simulink model "pacemaker_Integrated_modes_updated_AAI_VVI"  (R2023b)
settings: Solver=FixedStepAuto  StartTime=0.0  StopTime=10  FixedStep=1e-3  RelTol=1e-3  EnableMultiTasking=on
undefined symbols (not defined in the file): D0, D1, D10, D11, D12, D13, D2, D3, D4, D5, D6, D7, D8, D9, PTA0, PTA1, PTA2, PTB23, PTB9, PTC16, PTC17, PTC2, PTC3, PTC4, PTD0, PTD1, PTD2, PTD3
libraries: frdmk64flib x16
settings Model: ExtModeTrigDuration=5  Creator=sadeg  LastModifiedBy=ayush
settings OptimizationCC: EnhancedBackFolding=on  PassReuseOutputArgsThreshold=0  MaxStackSize=64  OptimizeBlockOrder=speed  DifferentSizesBufferReuse=on  OptimizationCustomize=off
settings DebuggingCC: ParameterTunabilityLossMsg=error
settings HardwareCC: ProdBitPerPointer=32  ProdBitPerSizeT=32  ProdBitPerPtrDiffT=32  ProdLargestAtomicInteger=Long  ProdLargestAtomicFloat=Double  ProdWordSize=32  ProdHWDeviceType=ARM Compatible->ARM Cortex  UseEmbeddedCoderFeatures=off
settings SFSimCC: MATLABDynamicMemAlloc=off
settings RTWCC: Description=Embedded Coder  SystemTargetFile=ert.tlc  HardwareBoard=NXP FRDM-K64F  TLCOptions="-aInlineSetEventsForThisBaseRateFcn=TLC_FALSE -aSuppressMultiTaskScheduler=TLC_FALSE  -aRateBasedStepFcn=0"  TemplateMakefile=ert_default_tmf  Toolchain=GNU Tools for ARM Embedded Processors
settings CodeAppCC: ForceParamTrailComments=on  OperatorAnnotations=on
settings ERTTargetCC: ERTCustomFileBanners=off  SupportContinuousTime=on  SupportNonInlinedSFcns=on  RemoveResetFunc=off  ModelStepFunctionPrototypeControlCompliant=off  ExtModeTransport=4  ExtModeMexFile=sendToCommService

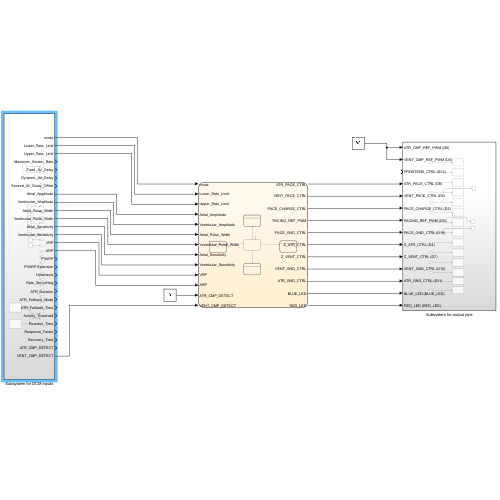
[thumbnail: Simulink's stored preview of the top-level diagram]
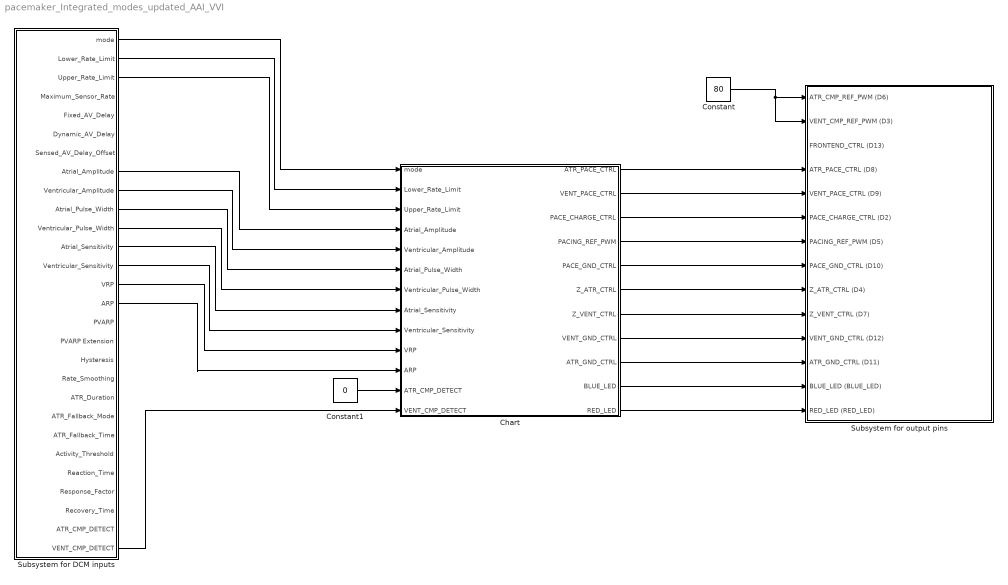
== system pacemaker_Integrated_modes_updated_AAI_VVI ==
  Chart : Stateflow chart  TreatAsAtomicUnit=on
      settings: PortSchema="{\"entries\":[{\"content\":{\"sides\":[{\"content\":{\"connectorIds\":[\"In13\",\"In1\",\"In2\",\"In3\",\"In5\",\"In4\",\"In6\",\"In7\",\"In8\",\"In10\",\"In9\",\"In12\",\"In11\"]},\"type\":\"ConnectorPlacement.EquallySpacedRectSide\",\"uuid\":\"4624e3e5-9266-4e51-8f1f-a7517f1382a8\"},{\"content\":{\"connectorIds\":[\"Out3\",\"Out4\",\"Out2\",\"Out5\",\"Out6\",\"Out7\",\"Out1\",\"Out8\",\"Out9\",\"Out10\",\"Out11\"],\"side\":\"RIGHT\"},\"type\":\"ConnectorPlacement.EquallySpacedRectSide\",\"uuid\":\"506810c9-9779-465d-935e-bf5d90de1bf6\"},{\"content\":{\"side\":\"TOP\"},\"type\":\"ConnectorPlacement.EquallySpacedRectSide\",\"uuid\":\"ef5dabc6-fa85-4901-94e2-5ef8203e9e04\"}]},\"type\":\"ConnectorPlacement.EquallySpacedConnector\",\"uuid\":\"5b51df89-7be9-413b-8f7d-b7db43a61802\"}],\"packageUris\":[\"http://schema.mathworks.com/mf0/Connector/R2020b\"],\"version\":\"1.0\"}"
  Constant : Constant  Value=80
  Constant1 : Constant  Value=0
  Subsystem for DCM inputs : Subsystem
  Subsystem for output pins : Subsystem
  wires:
  Constant/1 -> Subsystem for output pins/2(VENT_CMP_REF_PWM (D3)), Subsystem for output pins/1(ATR_CMP_REF_PWM (D6))
  Subsystem for DCM inputs/2(Lower_Rate_Limit) -> Chart/1(Lower_Rate_Limit)
  Subsystem for DCM inputs/3(Upper_Rate_Limit) -> Chart/2(Upper_Rate_Limit)
  Subsystem for DCM inputs/8(Atrial_Amplitude) -> Chart/3(Atrial_Amplitude)
  Subsystem for DCM inputs/10(Atrial_Pulse_Width) -> Chart/4(Atrial_Pulse_Width)
  Subsystem for DCM inputs/9(Ventricular_Amplitude) -> Chart/5(Ventricular_Amplitude)
  Subsystem for DCM inputs/11(Ventricular_Pulse_Width) -> Chart/6(Ventricular_Pulse_Width)
  Subsystem for DCM inputs/12(Atrial_Sensitivity) -> Chart/7(Atrial_Sensitivity)
  Subsystem for DCM inputs/13(Ventricular_Sensitivity) -> Chart/8(Ventricular_Sensitivity)
  Subsystem for DCM inputs/15(ARP) -> Chart/9(ARP)
  Subsystem for DCM inputs/14(VRP) -> Chart/10(VRP)
  Chart/1(Z_VENT_CTRL) -> Subsystem for output pins/10(Z_VENT_CTRL (D7))
  Chart/2(PACE_CHARGE_CTRL) -> Subsystem for output pins/6(PACE_CHARGE_CTRL (D2))
  Chart/3(ATR_PACE_CTRL) -> Subsystem for output pins/4(ATR_PACE_CTRL (D8))
  Chart/4(VENT_PACE_CTRL) -> Subsystem for output pins/5(VENT_PACE_CTRL (D9))
  Chart/5(PACING_REF_PWM) -> Subsystem for output pins/7(PACING_REF_PWM (D5))
  Chart/6(PACE_GND_CTRL) -> Subsystem for output pins/8(PACE_GND_CTRL (D10))
  Chart/7(Z_ATR_CTRL) -> Subsystem for output pins/9(Z_ATR_CTRL (D4))
  Chart/8(VENT_GND_CTRL) -> Subsystem for output pins/11(VENT_GND_CTRL (D12))
  Chart/9(ATR_GND_CTRL) -> Subsystem for output pins/12(ATR_GND_CTRL (D11))
  Subsystem for DCM inputs/1(mode) -> Chart/13(mode)
  Subsystem for DCM inputs/28(VENT_CMP_DETECT) -> Chart/11(VENT_CMP_DETECT)
  Constant1/1 -> Chart/12(ATR_CMP_DETECT)
  Chart/10(BLUE_LED) -> Subsystem for output pins/13(BLUE_LED (BLUE_LED))
  Chart/11(RED_LED) -> Subsystem for output pins/14(RED_LED (RED_LED))

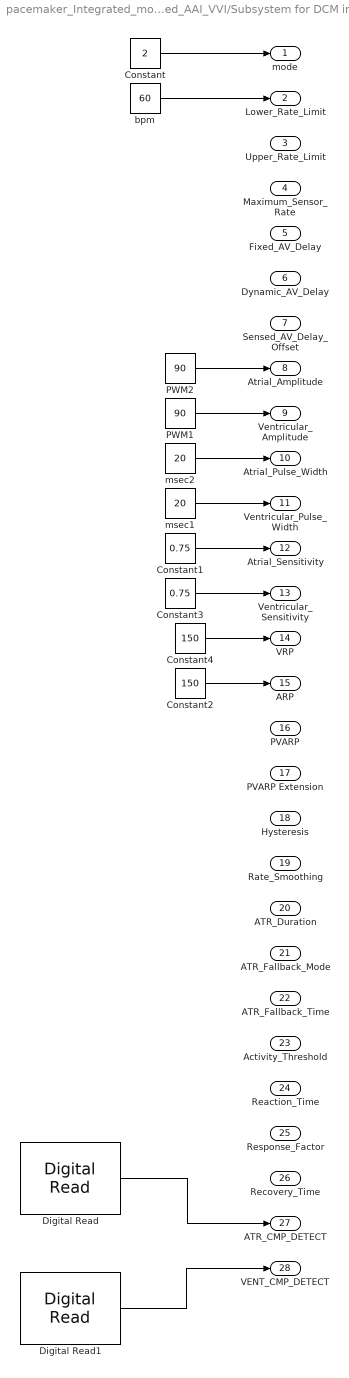
== system pacemaker_Integrated_modes_updated_AAI_VVI/Subsystem for DCM inputs ==
  Constant : Constant  Value=2
  Constant1 : Constant  Value=0.75
  Constant2 : Constant  Value=150
  Constant3 : Constant  Value=0.75
  Constant4 : Constant  Value=150
  Digital Read : frdmk64flib/Digital Read  Whichpin=PTC16 (D0)  SampleTime=-1
  Digital Read1 : frdmk64flib/Digital Read  Whichpin=PTC17 (D1)  SampleTime=-1
  PWM1 : Constant  Value=90
  PWM2 : Constant  Value=90
  bpm : Constant  Value=60
  msec1 : Constant  Value=20
  msec2 : Constant  Value=20
  mode : Outport
  Lower_Rate_Limit : Outport  Port=2
  Upper_Rate_Limit : Outport  Port=3
  Maximum_Sensor_Rate : Outport  Port=4
  Fixed_AV_Delay : Outport  Port=5
  Dynamic_AV_Delay : Outport  Port=6
  Sensed_AV_Delay_Offset : Outport  Port=7
  Atrial_Amplitude : Outport  Port=8
  Ventricular_Amplitude : Outport  Port=9
  Atrial_Pulse_Width : Outport  Port=10
  Ventricular_Pulse_Width : Outport  Port=11
  Atrial_Sensitivity : Outport  Port=12
  Ventricular_Sensitivity : Outport  Port=13
  VRP : Outport  Port=14
  ARP : Outport  Port=15
  PVARP : Outport  Port=16
  PVARP Extension : Outport  Port=17
  Hysteresis : Outport  Port=18
  Rate_Smoothing : Outport  Port=19
  ATR_Duration : Outport  Port=20
  ATR_Fallback_Mode : Outport  Port=21
  ATR_Fallback_Time : Outport  Port=22
  Activity_Threshold : Outport  Port=23
  Reaction_Time : Outport  Port=24
  Response_Factor : Outport  Port=25
  Recovery_Time : Outport  Port=26
  ATR_CMP_DETECT : Outport  Port=27
  VENT_CMP_DETECT : Outport  Port=28
  wires:
  bpm/1 -> Lower_Rate_Limit/1
  PWM1/1 -> Ventricular_Amplitude/1
  msec1/1 -> Ventricular_Pulse_Width/1
  Constant/1 -> mode/1
  PWM2/1 -> Atrial_Amplitude/1
  msec2/1 -> Atrial_Pulse_Width/1
  Constant1/1 -> Atrial_Sensitivity/1
  Constant2/1 -> ARP/1
  Constant3/1 -> Ventricular_Sensitivity/1
  Digital Read/1 -> ATR_CMP_DETECT/1
  Digital Read1/1 -> VENT_CMP_DETECT/1
  Constant4/1 -> VRP/1

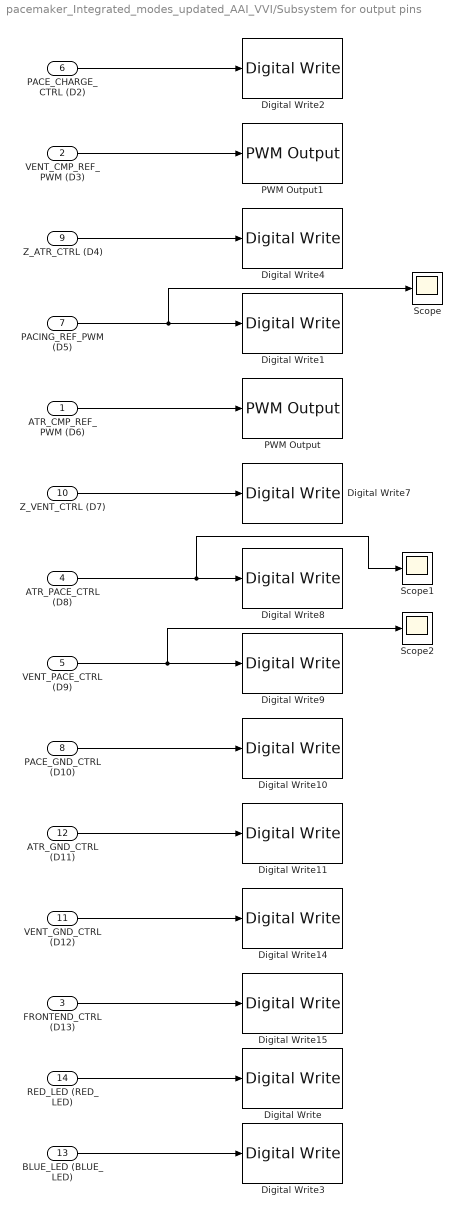
== system pacemaker_Integrated_modes_updated_AAI_VVI/Subsystem for output pins ==
  ATR_CMP_REF_PWM (D6) : Inport
  VENT_CMP_REF_PWM (D3) : Inport  Port=2
  FRONTEND_CTRL (D13) : Inport  Port=3
  ATR_PACE_CTRL (D8) : Inport  Port=4
  VENT_PACE_CTRL (D9) : Inport  Port=5
  PACE_CHARGE_CTRL (D2) : Inport  Port=6
  PACING_REF_PWM (D5) : Inport  Port=7
  PACE_GND_CTRL (D10) : Inport  Port=8
  Z_ATR_CTRL (D4) : Inport  Port=9
  Z_VENT_CTRL (D7) : Inport  Port=10
  VENT_GND_CTRL (D12) : Inport  Port=11
  ATR_GND_CTRL (D11) : Inport  Port=12
  BLUE_LED (BLUE_LED) : Inport  Port=13
  RED_LED (RED_LED) : Inport  Port=14
  Digital Write : frdmk64flib/Digital Write  Whichpin=RED_LED
  Digital Write1 : frdmk64flib/Digital Write  Whichpin=PTA2 (D5)
  Digital Write10 : frdmk64flib/Digital Write  Whichpin=PTD0 (D10)
  Digital Write11 : frdmk64flib/Digital Write  Whichpin=PTD2 (D11)
  Digital Write14 : frdmk64flib/Digital Write  Whichpin=PTD3 (D12)
  Digital Write15 : frdmk64flib/Digital Write  Whichpin=PTD1 (D13)
  Digital Write2 : frdmk64flib/Digital Write  Whichpin=PTB9 (D2)
  Digital Write3 : frdmk64flib/Digital Write  Whichpin=BLUE_LED
  Digital Write4 : frdmk64flib/Digital Write  Whichpin=PTB23 (D4)
  Digital Write7 : frdmk64flib/Digital Write  Whichpin=PTC3 (D7)
  Digital Write8 : frdmk64flib/Digital Write  Whichpin=PTA0 (D8)
  Digital Write9 : frdmk64flib/Digital Write  Whichpin=PTC4 (D9)
  PWM Output : frdmk64flib/PWM Output  Whichpin=PTC2 (D6)  InitialFrequency=2000  InitialDutyCycle=0
  PWM Output1 : frdmk64flib/PWM Output  Whichpin=PTA1 (D3)  InitialFrequency=2000  InitialDutyCycle=0
  Scope : Scope
  Scope1 : Scope
  Scope2 : Scope
  wires:
  PACE_CHARGE_CTRL (D2)/1 -> Digital Write2/1
  Z_ATR_CTRL (D4)/1 -> Digital Write4/1
  VENT_CMP_REF_PWM (D3)/1 -> PWM Output1/1
  PACING_REF_PWM (D5)/1 -> Digital Write1/1, Scope/1
  Z_VENT_CTRL (D7)/1 -> Digital Write7/1
  ATR_CMP_REF_PWM (D6)/1 -> PWM Output/1
  PACE_GND_CTRL (D10)/1 -> Digital Write10/1
  ATR_GND_CTRL (D11)/1 -> Digital Write11/1
  ATR_PACE_CTRL (D8)/1 -> Scope1/1, Digital Write8/1
  VENT_PACE_CTRL (D9)/1 -> Scope2/1, Digital Write9/1
  VENT_GND_CTRL (D12)/1 -> Digital Write14/1
  FRONTEND_CTRL (D13)/1 -> Digital Write15/1
  RED_LED (RED_LED)/1 -> Digital Write/1
  BLUE_LED (BLUE_LED)/1 -> Digital Write3/1

== stateflow chart pacemaker_Integrated_modes_updated_AAI_VVI/Chart ==
  state VOO
    note: VOO: Pace Ventrical at constant rate
    state Charging
      entry:
      PACING_REF_PWM = Ventricular_Amplitude;
      PACE_CHARGE_CTRL = 1;
      VENT_PACE_CTRL = 0;
      VENT_GND_CTRL = 1;
      PACE_GND_CTRL = 0;
      Z_VENT_CTRL = 0;
      ATR_PACE_CTRL = 0;
      ATR_GND_CTRL = 0;
      Z_ATR_CTRL = 0;
      %LED_RED = 0;
      %LED_BLUE = 1;
    state pacing
      entry:
      PACING_REF_PWM = Ventricular_Amplitude;
      PACE_CHARGE_CTRL = 0;
      VENT_PACE_CTRL = 1;
      VENT_GND_CTRL = 0;
      PACE_GND_CTRL = 1;
      Z_VENT_CTRL = 0;
      ATR_PACE_CTRL = 0;
      ATR_GND_CTRL = 0;
      Z_ATR_CTRL = 0;
      %LED_RED = 1;
      %LED_BLUE = 0;
    (default) -> VOO.Charging
    VOO.Charging -> pacing : [after((60000/Lower_Rate_Limit)- (Ventricular_Pulse_Width), msec)]
    pacing -> VOO.Charging : [after(Ventricular_Pulse_Width,msec)]
  state start
  state AAI
    state Pacing
      entry:
      PACING_REF_PWM = Atrial_Amplitude;
      PACE_CHARGE_CTRL=0;
      ATR_PACE_CTRL= 1;
      ATR_GND_CTRL= 0;
      PACE_GND_CTRL=1;
      Z_ATR_CTRL=0;
      RED_LED = 0
      BLUE_LED = 1
    state Charging_and_Sensing
      entry:
      PACING_REF_PWM = Atrial_Amplitude
      PACE_CHARGE_CTRL=1;
      ATR_PACE_CTRL= 0;
      ATR_GND_CTRL= 1;
      PACE_GND_CTRL=0;
      Z_ATR_CTRL=0;
      %FRONTEND_CTRL = 1;
      %ATR_CMP_REF_PWM = Atrial_Sensitivity;
      RED_LED = 1
      BLUE_LED = 0
    (default) -> Charging_and_Sensing
    Pacing -> Charging_and_Sensing : after(Atrial_Pulse_Width,msec)
    Charging_and_Sensing -> (junction 165) : after(ARP-Atrial_Pulse_Width, msec)
    (junction 165) -> Pacing [order 2] : after((60000/Lower_Rate_Limit)-ARP,msec)[ATR_CMP_DETECT == 0]
    (junction 165) -> Charging_and_Sensing [order 1] : [ATR_CMP_DETECT == 1]
  state AOO
    note: AOO: Pace Atrium at constant rate
    state Charging
      entry:
      PACING_REF_PWM = Atrial_Amplitude;
      PACE_CHARGE_CTRL = 1;
      ATR_PACE_CTRL = 0;
      ATR_GND_CTRL = 1;
      PACE_GND_CTRL = 0;
      Z_ATR_CTRL = 0;
      VENT_PACE_CTRL = 0;
      VENT_GND_CTRL = 0;
      Z_VENT_CTRL = 0;
      %LED_RED = 0;
      %LED_BLUE = 1;
    state Discharging
      entry:
      PACING_REF_PWM = Atrial_Amplitude;
      PACE_CHARGE_CTRL = 0;
      ATR_PACE_CTRL = 1;
      ATR_GND_CTRL = 0;
      PACE_GND_CTRL = 1;
      Z_ATR_CTRL = 0;
      VENT_PACE_CTRL = 0;
      VENT_GND_CTRL = 0;
      Z_VENT_CTRL = 0;
      %LED_RED = 1;
      %LED_BLUE = 0;
    (default) -> AOO.Charging
    AOO.Charging -> Discharging : [after((60000/Lower_Rate_Limit)- (Atrial_Pulse_Width), msec)]
    Discharging -> AOO.Charging : [after(Atrial_Pulse_Width,msec)]
  state VVI
    state Pacing1
      entry:
      PACING_REF_PWM = Ventricular_Amplitude;
      PACE_CHARGE_CTRL = 0;
      VENT_PACE_CTRL = 1;
      VENT_GND_CTRL = 0;
      PACE_GND_CTRL = 1;
      Z_VENT_CTRL = 0;
    state Charging_and_Sensing1
      entry:
      PACING_REF_PWM = Ventricular_Amplitude;
      PACE_CHARGE_CTRL = 1;
      VENT_PACE_CTRL = 0;
      VENT_GND_CTRL = 1;
      PACE_GND_CTRL = 0;
      Z_VENT_CTRL = 0;
      %FRONTEND_CTRL = 1;
      %VENT_CMP_REF_PWM = S_Amp;
    (default) -> Charging_and_Sensing1
    Pacing1 -> Charging_and_Sensing1 : [after(Ventricular_Pulse_Width,msec)]
    Charging_and_Sensing1 -> (junction 179) : after(VRP-Ventricular_Pulse_Width,msec)
    (junction 179) -> Pacing1 [order 2] : after((60000/Lower_Rate_Limit)-VRP,msec)[VENT_CMP_DETECT == 0]
    (junction 179) -> Charging_and_Sensing1 [order 1] : [VENT_CMP_DETECT == 1]
  start -> VOO [order 2] : [mode ==2]
  (default) -> start
  start -> AOO [order 1] : [mode ==1]
  start -> AAI [order 3] : [mode ==3]
  start -> VVI [order 4] : [mode==4]
  data: Lower_Rate_Limit input; Upper_Rate_Limit input; Atrial_Amplitude input; Atrial_Pulse_Width input; Ventricular_Amplitude input; Ventricular_Pulse_Width input; Z_VENT_CTRL output; PACE_CHARGE_CTRL output; ATR_PACE_CTRL output; VENT_PACE_CTRL output; PACING_REF_PWM output; PACE_GND_CTRL output; Z_ATR_CTRL output; VENT_GND_CTRL output; ATR_CMP_REF_PWM local; VENT_CMP_REF_PWM local; Atrial_Sensitivity input; Ventricular_Sensitivity input; ATR_GND_CTRL output; ARP input; VRP input; VENT_CMP_DETECT input; ATR_CMP_DETECT input; mode input; BLUE_LED output; RED_LED output
